simulink model "Tracking_Lane_Detection"  (R2017a)
settings: Solver=FixedStepDiscrete  StartTime=0.0  StopTime=inf  RelTol=1e-3  EnableMultiTasking=on
libraries: visiontransforms x2, visionanalysis x1, visionstatistics x1
settings Model: Creator=ChiChaChai  LastModifiedBy=ChiChaChai
settings SolverCC: PositivePriorityOrder=on  AutoInsertRateTranBlk=on
settings DataIOCC: SaveOutput=off  SaveTime=off
settings OptimizationCC: DefaultParameterBehavior=Inlined  UseDivisionForNetSlopeComputation=on  UseFloatMulNetSlope=on  InlineInvariantSignals=on  PassReuseOutputArgsAs=Individual arguments  ZeroExternalMemoryAtStartup=off  ZeroInternalMemoryAtStartup=off  NoFixptDivByZeroProtection=on  EfficientFloat2IntCast=on  LifeSpan=1  MaxStackSize=64
settings DebuggingCC: ParameterTunabilityLossMsg=error
settings HardwareCC: ProdBitPerPointer=32  ProdBitPerSizeT=32  ProdBitPerPtrDiffT=32  ProdLargestAtomicInteger=Long  ProdLargestAtomicFloat=Double  ProdWordSize=32  ProdHWDeviceType=ARM Compatible->ARM Cortex
settings ModelReferenceCC: PropagateVarSize=During execution
settings SFSimCC: MATLABDynamicMemAlloc=off
settings RTWCC: SystemTargetFile=ert.tlc  HardwareBoard=Raspberry Pi  TLCOptions="-aInlineSetEventsForThisBaseRateFcn=TLC_FALSE -aSuppressMultiTaskScheduler=TLC_FALSE  -aRateBasedStepFcn=0"  TemplateMakefile=ert_default_tmf  Description=Embedded Coder  GenerateReport=on  Toolchain=GNU GCC Raspberry Pi  IncludeHyperlinkInReport=on  LaunchReport=on  GenerateTraceInfo=on  GenerateTraceReport=on  GenerateTraceReportSl=on  GenerateTraceReportSf=on  GenerateTraceReportEml=on  GenerateCodeMetricsReport=on
settings CodeAppCC: ForceParamTrailComments=on  IgnoreCustomStorageClasses=off  OperatorAnnotations=on  SimulinkDataObjDesc=on  SFDataObjDesc=on  MATLABFcnDesc=on  CustomSymbolStrGlobalVar=rt$N$M  CustomSymbolStrType=$N$M  CustomSymbolStrFcn=$N$M$F  CustomSymbolStrMacro=$N$M  InsertBlockDesc=on  MATLABSourceComments=on
settings ERTTargetCC: IncludeMdlTerminateFcn=off  CombineSignalStateStructs=on  SupportAbsoluteTime=off  SupportComplex=off  SupportNonInlinedSFcns=on  SupportVariableSizeSignals=on  ExtMode=on  ExtModeMexArgs='192.168.1.228' 0 17725  InlinedParameterPlacement=NonHierarchical  ERTFilePackagingFormat=CompactWithDataFile

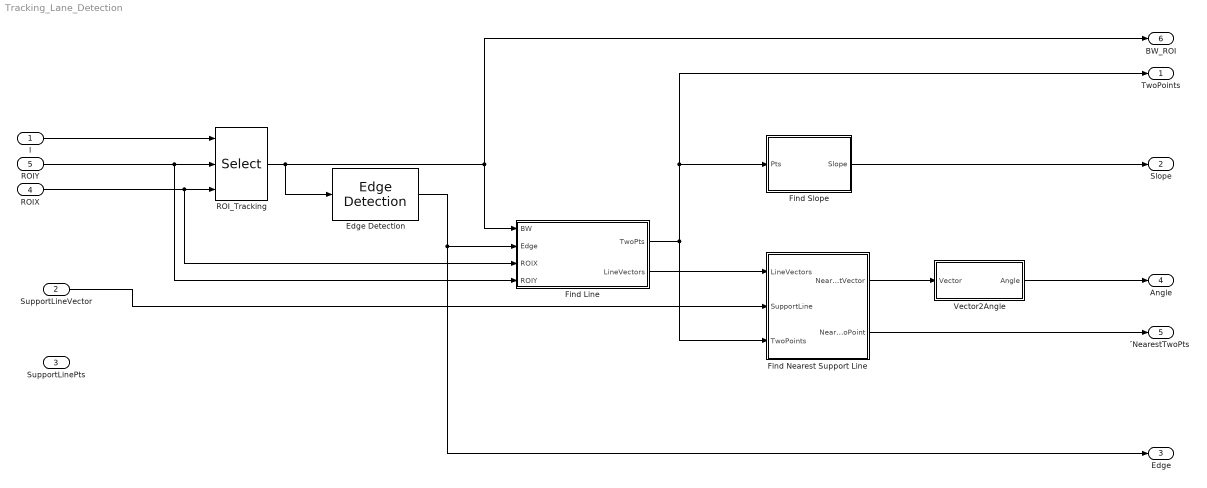
== system Tracking_Lane_Detection ==
  I : Inport  OutDataTypeStr=uint8  PortDimensions=[240 320]  SampleTime=[0.02,0]
  SupportLineVector : Inport  Port=2  OutDataTypeStr=double  PortDimensions=[1 2]
  SupportLinePts : Inport  Port=3  OutDataTypeStr=double  PortDimensions=4
  ROIX : Inport  Port=4  OutDataTypeStr=double  PortDimensions=281
  ROIY : Inport  Port=5  OutDataTypeStr=double  PortDimensions=31
  Edge Detection : visionanalysis/Edge Detection  method=Sobel  outputType=Binary image  userDefinedThreshold=off  thresholdSource=Input port  threshold=10  thresholdTuning=4  edgeThinning=on  threshold_canny=[0.25 0.60]  autoPercent=25  sigma=1  prodOutputMode=Binary point scaling  prodOutputWordLength=32  prodOutputFracLength=8  roundingMode=Floor  overflowMode=off
      settings: SourceProductName=Computer Vision System Toolbox  SourceProductBaseCode=VP
  Find Line : Subsystem
  Find Nearest Support Line : Subsystem
  Find Slope : Subsystem
  ROI_Tracking : Selector  NumberOfDimensions=2  InputPortWidth=3  IndexOptions=Index vector (port),Index vector (port)  Indices=[1 3],1  OutputSizes=1,1
  Vector2Angle : Subsystem
  TwoPoints : Outport  OutDataTypeStr=int32  PortDimensions=[5 4]  SampleTime=[0.020000000000000001,0]
      settings: VarSizeSig=Yes
  Slope : Outport  Port=2  OutDataTypeStr=double  PortDimensions=[5 1]  SampleTime=[0.020000000000000001,0]
      settings: VarSizeSig=Yes
  Edge : Outport  Port=3  OutDataTypeStr=boolean  PortDimensions=[31 281]  SampleTime=[0.020000000000000001,0]
  Angle : Outport  Port=4  OutDataTypeStr=double  PortDimensions=[1 1]  SampleTime=[0.02,0]
  ์NearestTwoPts : Outport  Port=5  OutDataTypeStr=int32  PortDimensions=[1 4]  SampleTime=[0.02,0]
  BW_ROI : Outport  Port=6  OutDataTypeStr=uint8  PortDimensions=[31 281]  SampleTime=[0.02,0]
  wires:
  Vector2Angle/1(Angle) -> Angle/1
  Find Line/1(TwoPts) -> Find Nearest Support Line/3(TwoPoints), Find Slope/1(Pts), TwoPoints/1
  ROIX/1 -> ROI_Tracking/3, Find Line/3(ROIX)
  Find Nearest Support Line/2(NearestTwoPoint) -> ์NearestTwoPts/1
  Find Nearest Support Line/1(NearestVector) -> Vector2Angle/1(Vector)
  Edge Detection/1 -> Find Line/2(Edge), Edge/1
  ROI_Tracking/1 -> BW_ROI/1, Find Line/1(BW), Edge Detection/1
  I/1 -> ROI_Tracking/1
  Find Line/2(LineVectors) -> Find Nearest Support Line/1(LineVectors)
  SupportLineVector/1 -> Find Nearest Support Line/2(SupportLine)
  Find Slope/1(Slope) -> Slope/1
  ROIY/1 -> ROI_Tracking/2, Find Line/4(ROIY)

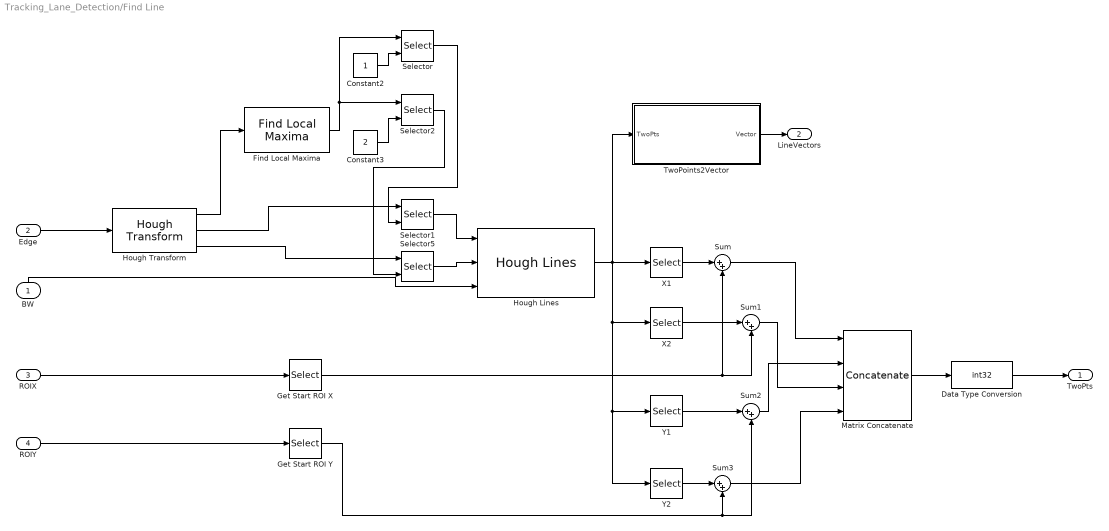
== system Tracking_Lane_Detection/Find Line ==
  BW : Inport
  Edge : Inport  Port=2
  ROIX : Inport  Port=3
  ROIY : Inport  Port=4
  Constant2 : Constant
  Constant3 : Constant  Value=2
  Data Type Conversion : DataTypeConversion  OutDataTypeStr=int32
  Find Local Maxima : visionstatistics/Find Local Maxima  num_peaks=5  nhood_size=[5 7]  src_thresh=Obsolete9b  src_thresh_inuse=Specify via dialog  threshold=10  inputIsHough=on  dt_peak=uint32  isOutVarDim=on  dt_count=uint32
      settings: SourceProductName=Computer Vision System Toolbox  SourceProductBaseCode=VP
  Get Start ROI X : Selector  InputPortWidth=281  IndexOptions=Index vector (dialog)  Indices=[1 ]  OutputSizes=1
  Get Start ROI Y : Selector  InputPortWidth=31  IndexOptions=Index vector (dialog)  Indices=[1 ]  OutputSizes=1
  Hough Lines : visiontransforms/Hough Lines  sineCompMethod=Trigonometric function  thetaRes=pi/180  firstCoeffMode=Specify word length  firstCoeffWordLength=16  firstCoeffFracLength=15  prodOutputMode=Binary point scaling  prodOutputWordLength=32  prodOutputFracLength=16  roundingMode=Nearest  overflowMode=on
      settings: SourceProductName=Computer Vision System Toolbox  SourceProductBaseCode=VP
  Hough Transform : visiontransforms/Hough Transform  theta_res=pi/180*8  rho_res=1  out_theta_rho=on  outdtmode=double  firstCoeffMode=Binary point scaling  firstCoeffWordLength=16  firstCoeffFracLength=14  secondCoeffMode=Binary point scaling  secondCoeffWordLength=32  secondCoeffFracLength=16  outputMode=Binary point scaling  outputWordLength=16  outputFracLength=0  accumMode=Binary point scaling  accumWordLength=32  accumFracLength=20  prodOutputMode=Binary point scaling  prodOutputWordLength=32  prodOutputFracLength=20  memoryMode=Binary point scaling  memoryWordLength=32  memoryFracLength=16  roundingMode=Nearest  overflowMode=on
      settings: SourceProductName=Computer Vision System Toolbox  SourceProductBaseCode=VP
  Matrix Concatenate : Concatenate  NumInputs=4  Mode=Multidimensional array  ConcatenateDimension=2
  Selector{,1..2,5} (4 alike) : Selector  NumberOfDimensions=2  InputPortWidth=3  IndexOptions=Select all,Index vector (port)  Indices=[1 3],1  OutputSizes=1,1
  Sum{,1..3} (4 alike) : Sum  Inputs=|++
  TwoPoints2Vector : MATLAB Function  TreatAsAtomicUnit=on
  X1 : Selector  NumberOfDimensions=2  InputPortWidth=3  IndexOptions=Select all,Index vector (dialog)  Indices=[1 3],1  OutputSizes=1,1
  X2 : Selector  NumberOfDimensions=2  InputPortWidth=3  IndexOptions=Select all,Index vector (dialog)  Indices=[1 3],3  OutputSizes=1,1
  Y1 : Selector  NumberOfDimensions=2  InputPortWidth=3  IndexOptions=Select all,Index vector (dialog)  Indices=[1 3],2  OutputSizes=1,1
  Y2 : Selector  NumberOfDimensions=2  InputPortWidth=3  IndexOptions=Select all,Index vector (dialog)  Indices=[1 3],4  OutputSizes=1,1
  TwoPts : Outport
  LineVectors : Outport  Port=2
  wires:
  Data Type Conversion/1 -> TwoPts/1
  Sum2/1 -> Matrix Concatenate/2
  Sum1/1 -> Matrix Concatenate/3
  Sum/1 -> Matrix Concatenate/1
  Matrix Concatenate/1 -> Data Type Conversion/1
  Sum3/1 -> Matrix Concatenate/4
  Y2/1 -> Sum3/1
  Y1/1 -> Sum2/1
  Get Start ROI Y/1 -> Sum2/2, Sum3/2
  X2/1 -> Sum1/1
  Get Start ROI X/1 -> Sum1/2, Sum/2
  X1/1 -> Sum/1
  ROIY/1 -> Get Start ROI Y/1
  ROIX/1 -> Get Start ROI X/1
  TwoPoints2Vector/1(Vector) -> LineVectors/1
  Edge/1 -> Hough Transform/1
  Hough Lines/1 -> X1/1, TwoPoints2Vector/1(TwoPts), Y1/1, Y2/1, X2/1
  Selector2/1 -> Selector5/2
  Constant3/1 -> Selector2/2
  Selector/1 -> Selector1/2
  Find Local Maxima/1 -> Selector/1, Selector2/1
  Constant2/1 -> Selector/2
  Hough Transform/3 -> Selector5/1
  Selector5/1 -> Hough Lines/2
  Hough Transform/2 -> Selector1/1
  Selector1/1 -> Hough Lines/1
  Hough Transform/1 -> Find Local Maxima/1
  BW/1 -> Hough Lines/3

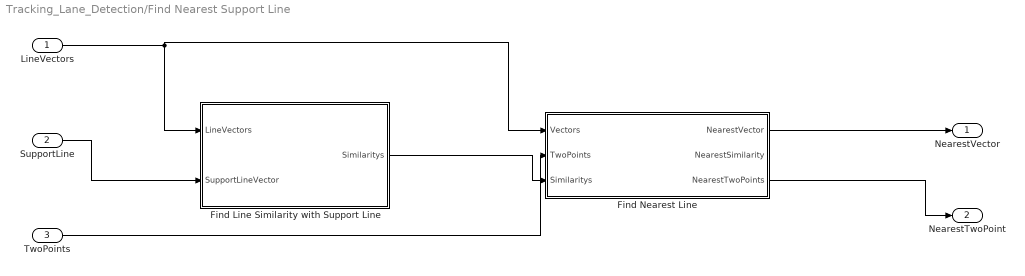
== system Tracking_Lane_Detection/Find Nearest Support Line ==
  LineVectors : Inport
  SupportLine : Inport  Port=2
  TwoPoints : Inport  Port=3
  Find Line Similarity with Support Line : MATLAB Function  TreatAsAtomicUnit=on
  Find Nearest Line : MATLAB Function  TreatAsAtomicUnit=on
  NearestVector : Outport  PortDimensions=[1 2]
  NearestTwoPoint : Outport  Port=2  PortDimensions=[1 4]
  wires:
  SupportLine/1 -> Find Line Similarity with Support Line/2(SupportLineVector)
  Find Line Similarity with Support Line/1(Similaritys) -> Find Nearest Line/3(Similaritys)
  LineVectors/1 -> Find Line Similarity with Support Line/1(LineVectors), Find Nearest Line/1(Vectors)
  Find Nearest Line/1(NearestVector) -> NearestVector/1
  Find Nearest Line/3(NearestTwoPoints) -> NearestTwoPoint/1
  TwoPoints/1 -> Find Nearest Line/2(TwoPoints)

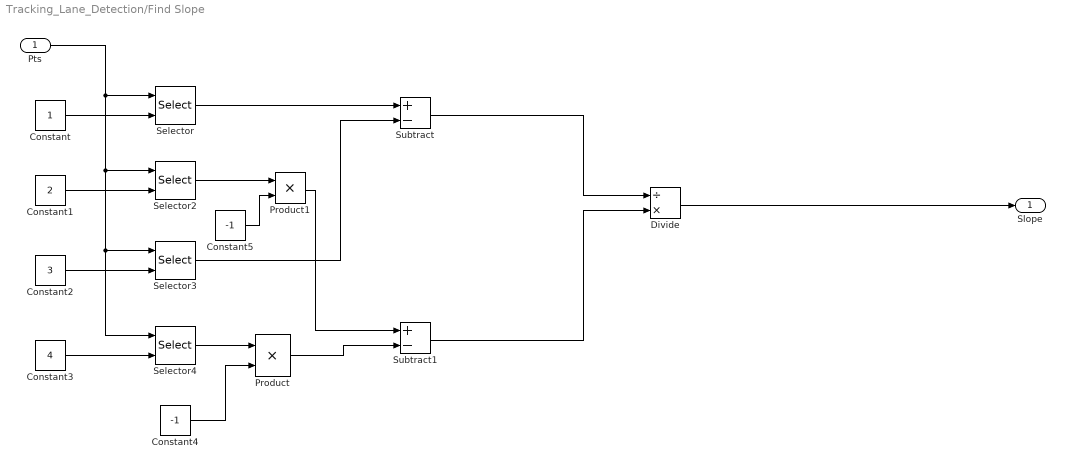
== system Tracking_Lane_Detection/Find Slope ==
  Pts : Inport
  Constant : Constant  OutDataTypeStr=uint8
  Constant1 : Constant  Value=2  OutDataTypeStr=uint8
  Constant2 : Constant  Value=3  OutDataTypeStr=uint8
  Constant3 : Constant  Value=4  OutDataTypeStr=uint8
  Constant4 : Constant  Value=-1
  Constant5 : Constant  Value=-1
  Divide : Product  Inputs=/*  OutDataTypeStr=double  RndMeth=Nearest
  Product : Product
  Product1 : Product
  Selector{,2..4} (4 alike) : Selector  NumberOfDimensions=2  InputPortWidth=3  IndexOptions=Select all,Index vector (port)  Indices=[1 3],1  OutputSizes=1,1
  Subtract : Sum  Inputs=+-
  Subtract1 : Sum  Inputs=+-
  Slope : Outport
  wires:
  Constant5/1 -> Product1/2
  Constant4/1 -> Product/2
  Product/1 -> Subtract1/2
  Product1/1 -> Subtract1/1
  Divide/1 -> Slope/1
  Subtract1/1 -> Divide/2
  Constant1/1 -> Selector2/2
  Constant2/1 -> Selector3/2
  Constant3/1 -> Selector4/2
  Subtract/1 -> Divide/1
  Constant/1 -> Selector/2
  Selector4/1 -> Product/1
  Selector2/1 -> Product1/1
  Selector/1 -> Subtract/1
  Selector3/1 -> Subtract/2
  Pts/1 -> Selector/1, Selector2/1, Selector4/1, Selector3/1

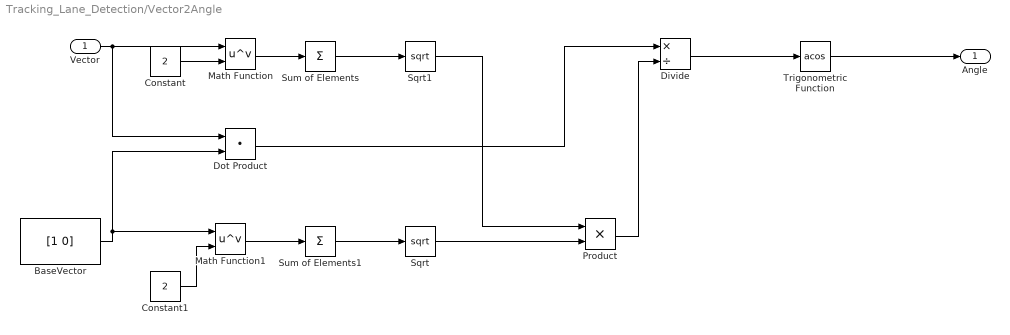
== system Tracking_Lane_Detection/Vector2Angle ==
  Vector : Inport
  BaseVector : Constant  Value=[1 0]  VectorParams1D=off
  Constant : Constant  Value=2
  Constant1 : Constant  Value=2
  Divide : Product  Inputs=*/
  Dot Product : DotProduct  InputSameDT=on  OutDataTypeStr=Inherit: Inherit via internal rule
  Math Function : Math  Operator=pow  SaturateOnIntegerOverflow=on
  Math Function1 : Math  Operator=pow  SaturateOnIntegerOverflow=on
  Product : Product
  Sqrt : Sqrt  SaturateOnIntegerOverflow=on
  Sqrt1 : Sqrt  SaturateOnIntegerOverflow=on
  Sum of Elements : Sum  Inputs=+
  Sum of Elements1 : Sum  Inputs=+
  Trigonometric Function : Trigonometry  Operator=acos
  Angle : Outport
  wires:
  Sqrt/1 -> Product/2
  Sqrt1/1 -> Product/1
  Sum of Elements1/1 -> Sqrt/1
  Sum of Elements/1 -> Sqrt1/1
  Constant1/1 -> Math Function1/2
  Constant/1 -> Math Function/2
  Trigonometric Function/1 -> Angle/1
  Divide/1 -> Trigonometric Function/1
  Product/1 -> Divide/2
  Dot Product/1 -> Divide/1
  Math Function1/1 -> Sum of Elements1/1
  Math Function/1 -> Sum of Elements/1
  BaseVector/1 -> Dot Product/2, Math Function1/1
  Vector/1 -> Dot Product/1, Math Function/1

== matlab function Tracking_Lane_Detection/Find Line/TwoPoints2Vector ==
  data: TwoPts input; Vector output size=[10 2]
function Vector = TwoPoints2Vector(TwoPts)
Vector = int32([ TwoPts(:,1)-TwoPts(:,3) -(TwoPts(:,2)-TwoPts(:,4))]);

== matlab function Tracking_Lane_Detection/Find Nearest Support Line/Find Line Similarity with Support Line ==
  data: LineVectors input; Similaritys output size=10; SupportLineVector input
function Similaritys= CosineSimilarity(LineVectors,SupportLineVector)
[m,n] = size(LineVectors);
LineVectors = double(LineVectors);

Similaritys = double(zeros(m,1));
%SupportLineVector = double([5 5]);
for i=1:m
    Similaritys(i) = (LineVectors(i,1)*SupportLineVector(1) + LineVectors(i,2)*SupportLineVector(2)) / (  sqrt(sum(LineVectors(i,:).^2)) * sqrt(sum(SupportLineVector(:).^2)) );
end

== matlab function Tracking_Lane_Detection/Find Nearest Support Line/Find Nearest Line ==
  data: Vectors input; TwoPoints input; NearestVector output; NearestSimilarity output size=1; Similaritys input; NearestTwoPoints output size=[1 4]
function [NearestVector,NearestSimilarity,NearestTwoPoints]= FindMostSimilarityLine(Vectors,TwoPoints,Similaritys)
Similaritys = abs(Similaritys);
[m,~]=size(Vectors);
NearestTwoPoints = int32([0 0 0 0]);
NearestSimilarity = double(0);
if m ~= 0
    NearestSimilarity = Similaritys(1);
    NearestVector = double(Vectors(1,1:2));

    for i = 1:m
        if Similaritys(i) > NearestSimilarity
            NearestSimilarity = Similaritys(i);
            NearestVector = double(Vectors(i,1:2));
            NearestTwoPoints = int32(TwoPoints(i,1:4));
        end
    end
else
    NearestVector = double([0 0]);
end
